simulink model "zad_no_2_b"  (R2017b)
settings: Solver=VariableStepAuto  StartTime=0.0  StopTime=10.0  RelTol=1e-3
undefined symbols (not defined in the file): Ini, Tp
settings Model: Creator=micha  LastModifiedBy=micha

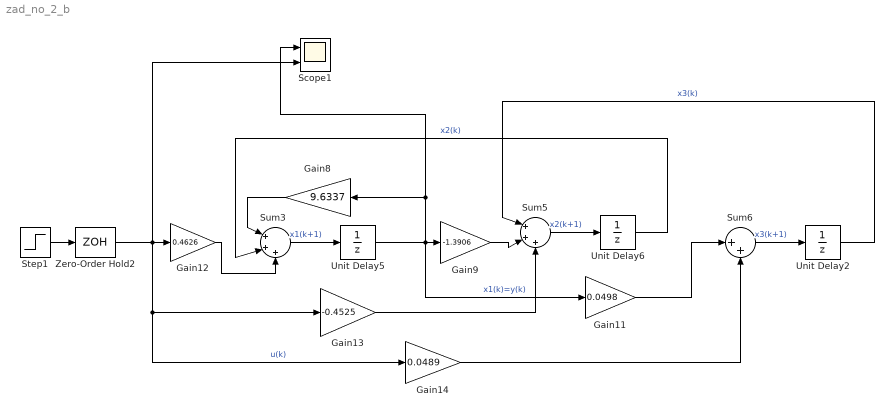
== system zad_no_2_b ==
  Gain11 : Gain  Gain=0.0498  ParamDataTypeStr=double
  Gain12 : Gain  Gain=0.4626  ParamDataTypeStr=double
  Gain13 : Gain  Gain=-0.4525  ParamDataTypeStr=double
  Gain14 : Gain  Gain=0.0489  ParamDataTypeStr=double
  Gain8 : Gain  Gain=9.6337  ParamDataTypeStr=double
  Gain9 : Gain  Gain=-1.3906  ParamDataTypeStr=double
  Scope1 : Scope  NumInputPorts=2
  Step1 : Step  SampleTime=0
  Sum3 : Sum  Inputs=|+++
  Sum5 : Sum  Inputs=|+++
  Sum6 : Sum  Inputs=|++
  Unit Delay2 : UnitDelay  InitialCondition=Ini  SampleTime=Tp
  Unit Delay5 : UnitDelay  InitialCondition=Ini  SampleTime=Tp
  Unit Delay6 : UnitDelay  InitialCondition=Ini  SampleTime=Tp
  Zero-Order Hold2 : ZeroOrderHold  SampleTime=Tp
  wires:
  Gain12/1 -> Sum3/3
  Gain11/1 -> Sum6/1
  Step1/1 -> Zero-Order Hold2/1
  Unit Delay5/1 -> Gain8/1, Scope1/1, Gain9/1, Gain11/1  "x1(k)=y(k)"
  Gain9/1 -> Sum5/2
  Zero-Order Hold2/1 -> Scope1/2, Gain12/1, Gain13/1, Gain14/1  "u(k)"
  Gain14/1 -> Sum6/2
  Gain13/1 -> Sum5/3
  Sum3/1 -> Unit Delay5/1  "x1(k+1)"
  Unit Delay6/1 -> Sum3/2  "x2(k)"
  Sum6/1 -> Unit Delay2/1  "x3(k+1)"
  Gain8/1 -> Sum3/1
  Unit Delay2/1 -> Sum5/1  "x3(k)"
  Sum5/1 -> Unit Delay6/1  "x2(k+1)"
